simulink model "proyecto_global_integrador_modelo"  (R2018a)
settings: Solver=VariableStepAuto  StartTime=0.0  StopTime=10.0  RelTol=1e-3
values from neighbouring files (symbols this model uses):
  b_eq = b_m + b_l/r^2    (= 1.5e-05)    [proyecto_global_integrador.m]
  C_ts = 1.091    [proyecto_global_integrador.m]
  J_eq = J_m + J_l/r^2    (= 5.65099476805e-06)    [proyecto_global_integrador.m]
  L_d = 6.6e-3    (= 0.0066)    [proyecto_global_integrador.m]
  L_ls = 0.8e-3    (= 0.0008)    [proyecto_global_integrador.m]
  L_q = 5.8e-3    (= 0.0058)    [proyecto_global_integrador.m]
  lambda_m = 0.01546    [proyecto_global_integrador.m]
  P_p = 3    [proyecto_global_integrador.m]
  r = 314.3008    [proyecto_global_integrador.m]
  R_s = 1.02    [polos_choreo_no_se_puede_robar_mas_con_esto.m]    (also in proyecto_global_integrador.m)
  R_tsamb = 55    [proyecto_global_integrador.m]
  T_ambmax = 40    [proyecto_global_integrador.m]
settings Model: Creator=gabrielq  LastModifiedBy=gabrielq

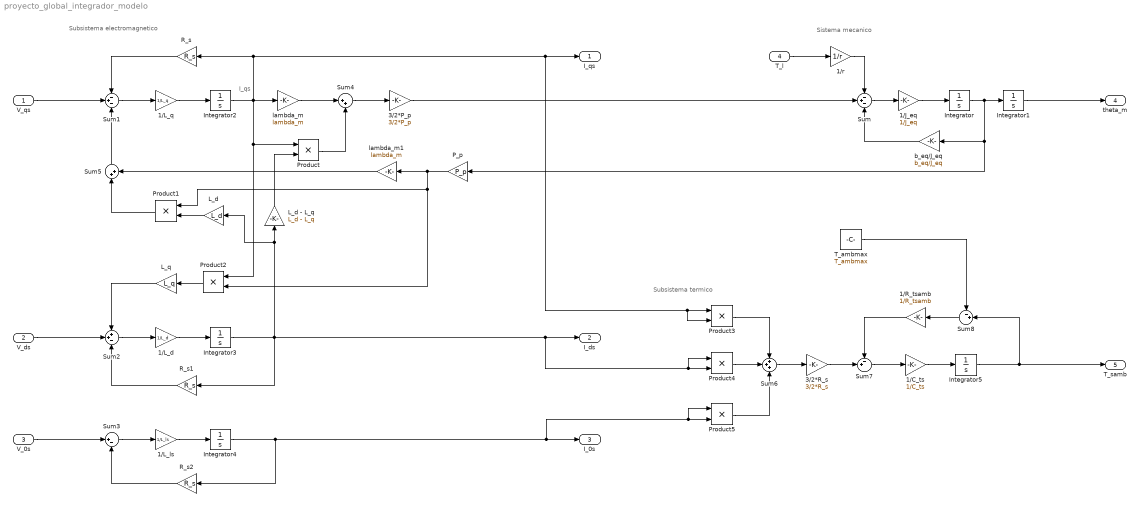
== system proyecto_global_integrador_modelo ==
  note: I_qs
  note: Subsistema termico
  note: Subsistema electromagnetico
  note: Sistema mecanico
  V_qs : Inport
  V_ds : Inport  Port=2
  V_0s : Inport  Port=3
  T_l : Inport  Port=4
  1/C_ts : Gain  Gain=1/C_ts
  1/J_eq : Gain  Gain=1/J_eq
  1/L_d : Gain  Gain=1/L_d
  1/L_ls : Gain  Gain=1/L_ls
  1/L_q : Gain  Gain=1/L_q
  1/R_tsamb : Gain  Gain=1/R_tsamb
  1/r : Gain  Gain=1/r
  3/2*P_p : Gain  Gain=3/2*P_p
  3/2*R_s : Gain  Gain=3/2*R_s
  Integrator{,1..5} (6 alike) : Integrator
  L_d : Gain  Gain=L_d
  L_d - L_q : Gain  Gain=L_d - L_q
  L_q : Gain  Gain=L_q
  P_p : Gain  Gain=P_p
  Product{,1..5} (6 alike) : Product
  R_s : Gain  Gain=R_s
  R_s1 : Gain  Gain=R_s
  R_s2 : Gain  Gain=R_s
  Sum : Sum  Inputs=-+-
  Sum1 : Sum  Inputs=-+-
  Sum2 : Sum  Inputs=++-
  Sum3 : Sum  Inputs=|+-
  Sum4 : Sum  Inputs=|++
  Sum5 : Sum  Inputs=|++
  Sum6 : Sum  Inputs=+++
  Sum7 : Sum  Inputs=-+|
  Sum8 : Sum  Inputs=-+|
  T_ambmax : Constant  Value=T_ambmax
  b_eq/J_eq : Gain  Gain=b_eq/J_eq
  lambda_m : Gain  Gain=lambda_m
  lambda_m1 : Gain  Gain=lambda_m
  I_qs : Outport
  I_ds : Outport  Port=2
  I_0s : Outport  Port=3
  theta_m : Outport  Port=4  SignalName=theta_m
  T_samb : Outport  Port=5
  wires:
  T_l/1 -> 1/r/1
  1/r/1 -> Sum/1
  Sum/1 -> 1/J_eq/1
  1/J_eq/1 -> Integrator/1
  Integrator/1 -> b_eq/J_eq/1, P_p/1, Integrator1/1
  b_eq/J_eq/1 -> Sum/3
  V_qs/1 -> Sum1/2
  V_ds/1 -> Sum2/2
  Sum1/1 -> 1/L_q/1
  R_s/1 -> Sum1/1
  1/L_q/1 -> Integrator2/1
  lambda_m/1 -> Sum4/1
  Sum4/1 -> 3/2*P_p/1
  3/2*P_p/1 -> Sum/2
  Product/1 -> Sum4/2
  Sum2/1 -> 1/L_d/1
  1/L_d/1 -> Integrator3/1
  L_d - L_q/1 -> Product/2
  R_s1/1 -> Sum2/3
  L_d/1 -> Product1/2
  Product1/1 -> Sum5/1
  lambda_m1/1 -> Sum5/2
  Sum5/1 -> Sum1/3
  P_p/1 -> lambda_m1/1, Product2/2, Product1/1
  L_q/1 -> Sum2/1
  Product2/1 -> L_q/1
  V_0s/1 -> Sum3/1
  Sum3/1 -> 1/L_ls/1
  R_s2/1 -> Sum3/2
  1/L_ls/1 -> Integrator4/1
  Integrator4/1 -> R_s2/1, Product5/1, Product5/2, I_0s/1
  Integrator1/1 -> theta_m/1
  Integrator2/1 -> Product/1, Product2/1, Product3/2, Product3/1, I_qs/1, R_s/1, lambda_m/1
  Integrator3/1 -> Product4/2, Product4/1, I_ds/1, R_s1/1, L_d/1, L_d - L_q/1
  Product3/1 -> Sum6/1
  Product4/1 -> Sum6/2
  Product5/1 -> Sum6/3
  Sum6/1 -> 3/2*R_s/1
  Sum7/1 -> 1/C_ts/1
  1/C_ts/1 -> Integrator5/1
  Integrator5/1 -> Sum8/2, T_samb/1
  3/2*R_s/1 -> Sum7/2
  Sum8/1 -> 1/R_tsamb/1
  T_ambmax/1 -> Sum8/1
  1/R_tsamb/1 -> Sum7/1
